simulink model "untitled"  (R2026a)
settings: Solver=VariableStepAuto
settings DataIOCC: TimeSaveName=t
settings DebuggingCC: ArtificialAlgebraicLoopMsg=none  MaxConsecutiveZCsMsg=none

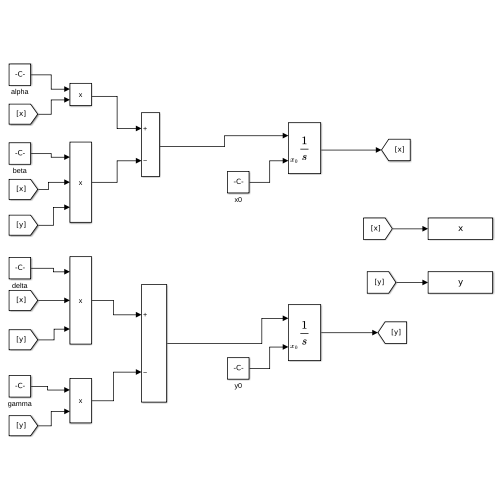
[thumbnail: Simulink's stored preview of the top-level diagram]
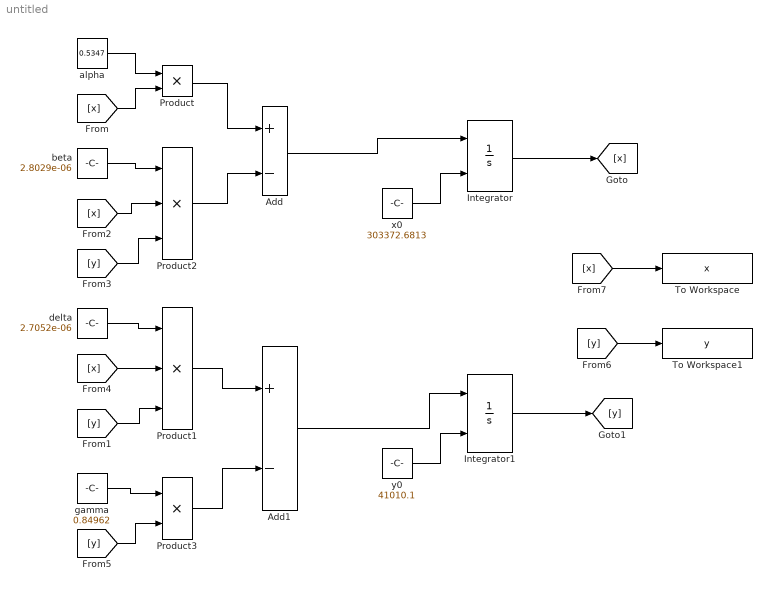
== system untitled ==
  Add : Sum  Inputs=+-
  Add1 : Sum  Inputs=+-
  Integrator : Integrator  InitialConditionSource=external
  Integrator1 : Integrator  InitialConditionSource=external
  Product : Product
  Product1 : Product  Inputs=3
  Product2 : Product  Inputs=3
  Product3 : Product
  To Workspace : ToWorkspace  VariableName=x  SampleTime=-1
  To Workspace1 : ToWorkspace  VariableName=y  SampleTime=-1
  alpha : Constant  Value=0.5347
  beta : Constant  Value=2.8029e-06
  delta : Constant  Value=2.7052e-06
  gamma : Constant  Value=0.84962
  x0 : Constant  Value=303372.6813
  y0 : Constant  Value=41010.1
  wires:
  x0/1 -> Integrator/2
  y0/1 -> Integrator1/2
  Add/1 -> Integrator/1
  Add1/1 -> Integrator1/1
  Integrator/1 -> [x]
  Integrator1/1 -> [y]
  alpha/1 -> Product/1
  [x] -> Product/2
  Product/1 -> Add/1
  beta/1 -> Product2/1
  [x] -> Product2/2
  Product2/1 -> Add/2
  [y] -> Product2/3
  delta/1 -> Product1/1
  [x] -> Product1/2
  [y] -> Product1/3
  Product1/1 -> Add1/1
  gamma/1 -> Product3/1
  [y] -> Product3/2
  Product3/1 -> Add1/2
  [x] -> To Workspace/1
  [y] -> To Workspace1/1
